simulink model "Rocky_model"  (R2024b)
settings: Solver=VariableStepAuto  StartTime=0.0  StopTime=20  RelTol=1e-3
model workspace (MAT data in the model file):
  C_i = 1
settings Model: Creator=jliu3  LastModifiedBy=jliu3

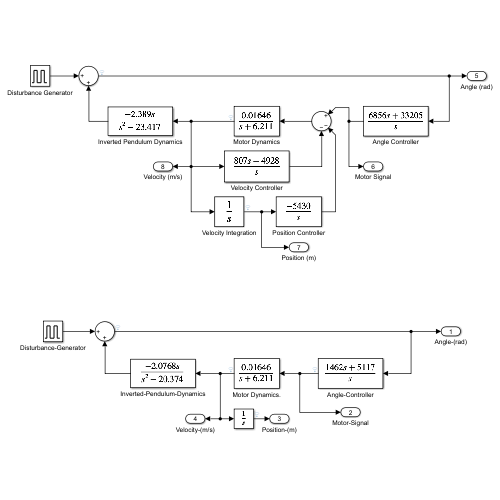
[thumbnail: Simulink's stored preview of the top-level diagram]
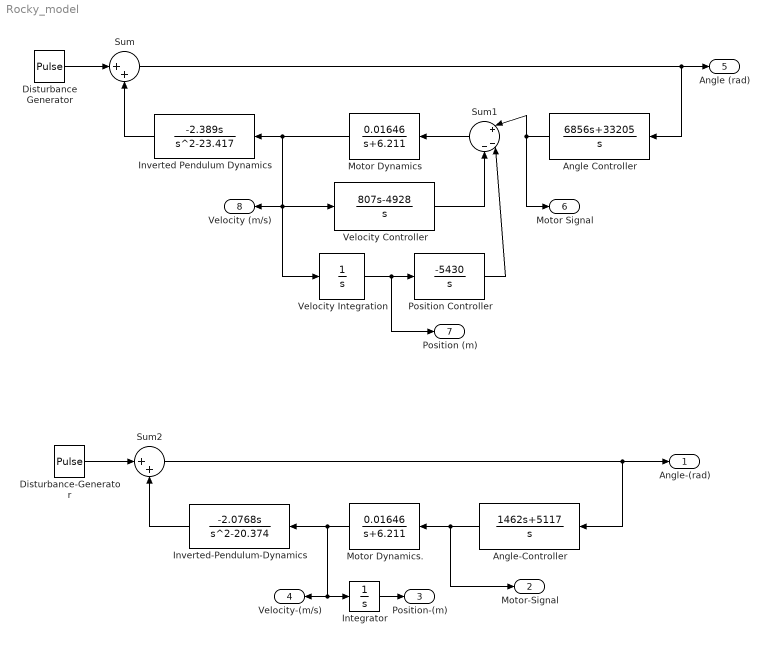
== system Rocky_model ==
  Angle Controller : TransferFcn  Numerator=[6856 33205]  Denominator=[1 0]
  Angle-Controller : TransferFcn  Numerator=[1462 5117]  Denominator=[1 0]
  Disturbance Generator : DiscretePulseGenerator  PulseType=Time based  Amplitude=0.3  Period=5  PulseWidth=0.1
  Disturbance-Generator : DiscretePulseGenerator  PulseType=Time based  Amplitude=0.3  Period=5  PulseWidth=0.1
  Integrator : Integrator
  Inverted Pendulum Dynamics : TransferFcn  Numerator=[-2.389 0]  Denominator=[1 0 -23.417]
  Inverted-Pendulum-Dynamics : TransferFcn  Numerator=[-2.0768 0]  Denominator=[1 0 -20.374]
  Motor Dynamics : TransferFcn  Numerator=[0.01646]  Denominator=[1 6.211]
  Motor Dynamics. : TransferFcn  Numerator=[0.01646]  Denominator=[1 6.211]
  Position Controller : TransferFcn  Numerator=-5430  Denominator=[1 0]
  Sum : Sum  Inputs=|++
  Sum1 : Sum  Inputs=|+|--
  Sum2 : Sum  Inputs=|++
  Velocity Controller : TransferFcn  Numerator=[807 -4928]  Denominator=[1 0]
  Velocity Integration : Integrator
  Angle-(rad) : Outport
  Motor-Signal : Outport  Port=2
  Position-(m) : Outport  Port=3
  Velocity-(m/s) : Outport  Port=4
  Angle (rad) : Outport  Port=5
  Motor Signal : Outport  Port=6
  Position (m) : Outport  Port=7
  Velocity (m/s) : Outport  Port=8
  wires:
  Sum/1 -> Angle Controller/1, Angle (rad)/1
  Inverted Pendulum Dynamics/1 -> Sum/2
  Disturbance Generator/1 -> Sum/1
  Velocity Controller/1 -> Sum1/3
  Sum1/1 -> Motor Dynamics/1
  Motor Dynamics/1 -> Inverted Pendulum Dynamics/1, Velocity Integration/1, Velocity (m/s)/1, Velocity Controller/1
  Velocity Integration/1 -> Position (m)/1, Position Controller/1
  Position Controller/1 -> Sum1/2
  Angle Controller/1 -> Motor Signal/1, Sum1/1
  Inverted-Pendulum-Dynamics/1 -> Sum2/2
  Sum2/1 -> Angle-(rad)/1, Angle-Controller/1
  Motor Dynamics./1 -> Inverted-Pendulum-Dynamics/1, Velocity-(m/s)/1, Integrator/1
  Disturbance-Generator/1 -> Sum2/1
  Angle-Controller/1 -> Motor-Signal/1, Motor Dynamics./1
  Integrator/1 -> Position-(m)/1
